simulink model "ng_pv_dynamic_dbus_p_1_sm_ng"  (Simulink 8.8)
settings: Solver=ode4  StartTime=0.0  StopTime=inf  FixedStep=0.000125  RelTol=1e-3  EnableMultiTasking=on
PreLoadFcn:
  | Ts=125e-6;Core_Num = 0; np=1; nq=1; Vmin=.9;
PostLoadFcn:
  | Ts=125e-6;Core_Num = 0; np=1; nq=1; Vmin=.9;
InitFcn:
  | Ts=125e-6;Core_Num = 0; np=1; nq=1; Vmin=.9;
undefined symbols (not defined in the file or in its folder): another_event_name, DiscIntNeverNeededParam, I, j, Left, my_event_name, Right, type, V, X
libraries: powerlib x316, simulink_extras x78, powerlib_meascontrol x47, ssn_lib x9, opal_lib x5, powerlib_extras x3, simulink x3, artemis x1, rtio_opalrt_ml605ex1 x1, rtlab x1, rtio_spectracom x1
(part 6 of 11)

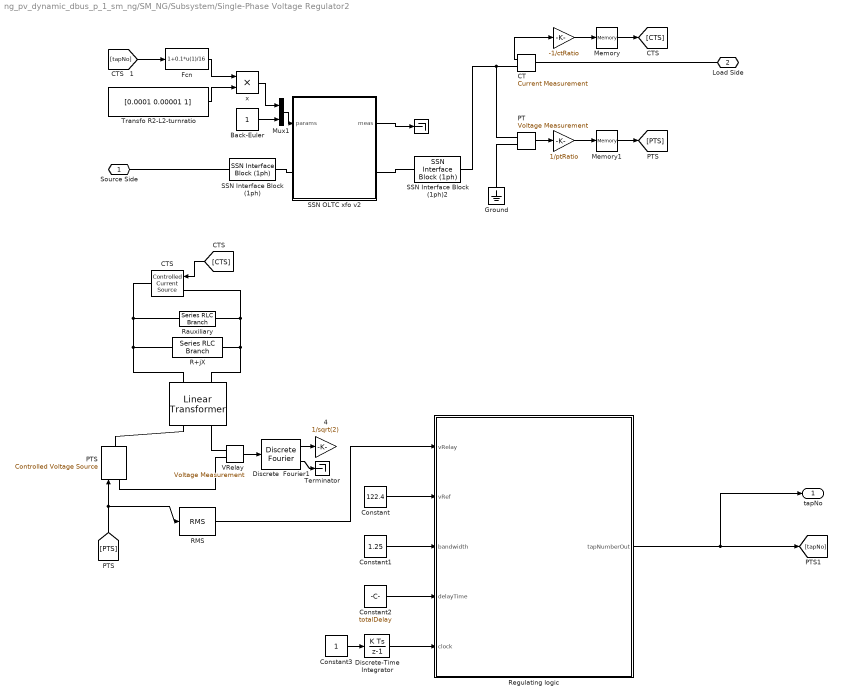
== system ng_pv_dynamic_dbus_p_1_sm_ng/SM_NG/Subsystem/Single-Phase Voltage Regulator2 ==
  " " : Gain  Gain=-1/ctRatio
  "   " : Terminator
  "    " : Gain  Gain=1/ptRatio
  "        " : powerlib/Elements/Linear Transformer  UNITS=SI  NominalPower=[pNom fNom]  winding1=[vNom/ptRatio 1.152e-007 1.2223e-008]  winding2=[vNom/ptRatio 1.152e-007 1.2223e-008]  ThreeWindings=off  winding3=[3.15e+005 0.7938 0.084225]  RmLm=[1.3824e+005 366.69]  Measurements=None  DataType=on
  "    4" : Gain  Gain=1/sqrt(2)
  Back-Euler : Constant
  CT : powerlib/Measurements/Current Measurement  PhasorSimulation=off  OutputType=Complex  PSBequivalent=0
  "CTS  " : powerlib/Electrical Sources/Controlled Current Source  Initialize=on  Source_Type=AC  Amplitude=0  Phase=0  Frequency=0  Measurements=None
  Constant : Constant  Value=122.4
  Constant1 : Constant  Value=1.25
  Constant2 : Constant  Value=totalDelay
  Constant3 : Constant
  Discrete  Fourier1 : powerlib_extras/Discrete Measurements/Discrete  Fourier  Freq=fNom  n=1  Par_Init=[0 0]  Ts=Ts
  Discrete-Time Integrator : DiscreteIntegrator  SampleTime=-1  ICPrevOutput=DiscIntNeverNeededParam  ICPrevScaledInput=DiscIntNeverNeededParam
  Fcn : Fcn  Expr=1+0.1*u(1)/16
  Ground : powerlib/Elements/Ground  LConnTagsString=a
  Memory : Memory
  Memory1 : Memory
  Mux1 : Mux  Inputs=2
  PT : powerlib/Measurements/Voltage Measurement  PhasorSimulation=off  OutputType=Complex  PSBequivalent=0
  "PTS  " : powerlib/Electrical Sources/Controlled Voltage Source  Initialize=on  Source_Type=AC  Amplitude=0  Phase=0  Frequency=0  Measurements=None
  R+jX : powerlib/Elements/Series RLC Branch  LConnTagsString=__new0  RConnTagsString=__new0  BranchType=RL  Resistance=r  Inductance=x / (2*pi*fNom)  SetiL0=off  InitialCurrent=0  Capacitance=1e-6  Setx0=off  InitialVoltage=0  Measurements=None
  RMS : powerlib_meascontrol/Measurements/RMS  TrueRMS=on  Freq=60  RMSInit=120  Ts=Ts
  Rauxiliary : powerlib/Elements/Series RLC Branch  LConnTagsString=__new0  RConnTagsString=__new0  BranchType=R  Resistance=1e3  Inductance=1.6 / (120*pi)  SetiL0=off  InitialCurrent=0  Capacitance=1e-6  Setx0=off  InitialVoltage=0  Measurements=None
  Regulating logic : MATLAB Function  TreatAsAtomicUnit=on
  SSN Interface Block (1ph) : ssn_lib/SSN Interface Block (1ph)  nb_phase=1  nb_port=2  p1_type=V-type(Left)  p2_type=X-type(Right)  p3_type=V-type(Left)  p4_type=V-type(Left)  p5_type=V-type(Left)  p6_type=V-type(Left)  p7_type=V-type(Left)  p8_type=V-type(Left)  p9_type=V-type(Left)  p10_type=V-type(Left)  p11_type=V-type(Left)  p12_type=V-type(Left)  p13_type=V-type(Left)  p14_type=V-type(Left)  p15_type=V-type(Left)  p16_type=V-type(Left)  I_port_shunt_resistance=1e9
  SSN Interface Block (1ph)2 : ssn_lib/SSN Interface Block (1ph)  nb_phase=1  nb_port=2  p1_type=X-type(Left)  p2_type=I-type(Right)  p3_type=X-type(Left)  p4_type=V-type (Right)  p5_type=V-type(Left)  p6_type=V-type(Left)  p7_type=V-type(Left)  p8_type=V-type(Left)  p9_type=V-type(Left)  p10_type=V-type(Left)  p11_type=V-type(Left)  p12_type=V-type(Left)  p13_type=V-type(Left)  p14_type=V-type(Left)  p15_type=V-type(Left)  p16_type=V-type(Left)  I_port_shunt_resistance=1e9
  SSN OLTC xfo v2 : Subsystem  AncestorBlock=artemis/SSN/SSN OLTC/SSN OLTC xfo v2  mask(Norton-Type External Nodal Subsystem){nnode=2, taggg=081xa09bxd1beaba51875, conntype=2 ports, RLpri=[1e-4 1e-5], Rcore=10000, ensat=on, Lcore=1000, Lsat=1000, phisat=1e8, Ts=Ts}
      mask prompts: nnode "Number of Electric nodes"; taggg "Unique Tag Identifier (automatic)"; conntype "Connection type"; RLpri "Primary winding resistance and inductance ([Ohms H])"; Rcore "Core Resistance (Ohms)"; ensat "Enable Saturation"; Lcore "Unsaturated magnetisation inductance (H)"; Lsat "Saturated magnetisation inductance (H)"; phisat "Flux saturation threshold (Weber)"; Ts "Sample Time (s)"
      mask help:
      | Continuously-variable On-Load Tapped Transformer (OLTC) (SSN Custom model)
      |
      | This block implements a 2 winding OLTC saturable transformer in SSN.
      | The model has a variable secondary inductance and resistance as well as turn-ratio.
      | The secondary winding is on the side marked with 'TAP'
      |
      | Mask parameters:
      |    Unique Tag Identifier: unique tag required by SSN to recknonize SSN external models
      |    Primary winding resistance and inductance ([Ohms H])
      |    Core Resistance (Ohms)
      |    Unsaturated magnetisation inductance (H): unsaturated core magnetization inductance
      |    Saturated magnetisation inductance (H): local inductance of the core in the saturated region
      |    Flux saturation threshold (Weber): flux saturation point
      |
      | Signal parameters:
      |
      | Signal inputs:
      |    1st sig: secondary winding resistance (Ohms)
      |    2nd sig: secondary winding inductance (H)
      |    3rd sig: transformer turn ratio k (V_secondary_tapped=k*V_primary)
      |    4th sig:  when set to 1, uses the Backward Euler method for solver. This can be used dynamically during simulation for example to damp numerical oscillations after switching events or after tap changes.
      |
      | Signals ouputs:
      |    1st signal: primary input current (A)
      |    2nd signal: secondary winding current (A)
      |    3rd signal: transformer flux (Wb)
      |
      | Saturation characteristic:
      |          flux
      |             ^              2
      |             |      1       *   <--- slope between point1 and point2 is Lsaturated
      |  phisat  |-----*  <---  this is the knee of flux=f(imag)
      |             |
      |             |
      |             |  <-----slope between origin and point1 is Lunsaturated
      |             *-------------------> imag
      mask init: same as ng_pv_dynamic_dbus_p_1_sm_ng/SM_NG/Subsystem/Single-Phase Voltage Regulator1/SSN OLTC xfo v2
      settings: CopyFcn=|
      | str=tempname;
      | str=strrep(str(end-20:end),'_','x');
      | set_param(gcb,'taggg',str);
      | set_param(gcb,'LinkStatus','inactive');
      mask Help: eval('open SSN_OLTC.pdf;');
      mask TypeOptions conntype: 4 ports | 3 ports (primary grounded) | 3 ports (tapped secondary grounded) | 2 ports
      mask Callback conntype:
      | bloc=gcb;
      | conntyp=get_param(bloc,'conntype');
      | nn=fts6_xfo_port_cb(bloc,conntyp);
      | set_param(bloc,'nnode',nn);
      mask Display:
      | plot(a1,a2,a3,a4,b1,b2,b3,b4,c1,c2,c3,c4,c5,c6,c7,c8,c9,c10,c11,c12,c13,c14,c15,c16);
      | color('blue');
      | plot(d1,d2,d3,d4,d5,d6,d7,d8,d9,d10);
  Terminator : Terminator
  Transfo R2-L2-turnratio : Constant  Value=[0.0001 0.00001 1]
  VRelay : powerlib/Measurements/Voltage Measurement  PhasorSimulation=off  OutputType=Complex  PSBequivalent=0
  x : Product  RndMeth=Zero
  Source Side : PMIOPort  Port=1  Side=Left
  Load Side : PMIOPort  Port=2  Side=Right
  tapNo : Outport
  wires:
  CT/1 -> " "/1
  " "/1 -> Memory/1
  PT/1 -> "    "/1
  "    "/1 -> Memory1/1
  [CTS] -> "CTS  "/1
  [PTS] -> RMS/1, "PTS  "/1
  VRelay/1 -> Discrete  Fourier1/1
  Discrete  Fourier1/1 -> "    4"/1
  Discrete-Time Integrator/1 -> Regulating logic/5(clock)
  Regulating logic/1(tapNumberOut) -> [tapNo], tapNo/1
  Constant/1 -> Regulating logic/2(vRef)
  Constant1/1 -> Regulating logic/3(bandwidth)
  Constant2/1 -> Regulating logic/4(delayTime)
  Memory/1 -> [CTS]
  Memory1/1 -> [PTS]
  Discrete  Fourier1/2 -> Terminator/1
  Back-Euler/1 -> Mux1/2
  Transfo R2-L2-turnratio/1 -> x/2
  x/1 -> Mux1/1
  Fcn/1 -> x/1
  [tapNo] -> Fcn/1
  Constant3/1 -> Discrete-Time Integrator/1
  RMS/1 -> Regulating logic/1(vRelay)
  Mux1/1 -> SSN OLTC xfo v2/1(params)
  SSN OLTC xfo v2/1(meas) -> "   "/1
  connections:
  R+jX/LConn1 -- "        "/LConn1 -- "CTS  "/RConn1 -- Rauxiliary/LConn1
  R+jX/RConn1 -- "        "/LConn2 -- "CTS  "/LConn1 -- Rauxiliary/RConn1
  "PTS  "/RConn1 -- "        "/RConn1
  "        "/RConn2 -- VRelay/LConn1
  PT/LConn1 -- CT/RConn1 -- SSN Interface Block (1ph)2/RConn1
  PT/LConn2 -- Ground/LConn1
  VRelay/LConn2 -- "PTS  "/LConn1
  Load Side/RConn1 -- CT/LConn1
  SSN Interface Block (1ph)/RConn1 -- SSN OLTC xfo v2/LConn1
  SSN Interface Block (1ph)2/LConn1 -- SSN OLTC xfo v2/RConn1
  SSN Interface Block (1ph)/LConn1 -- Source Side/RConn1

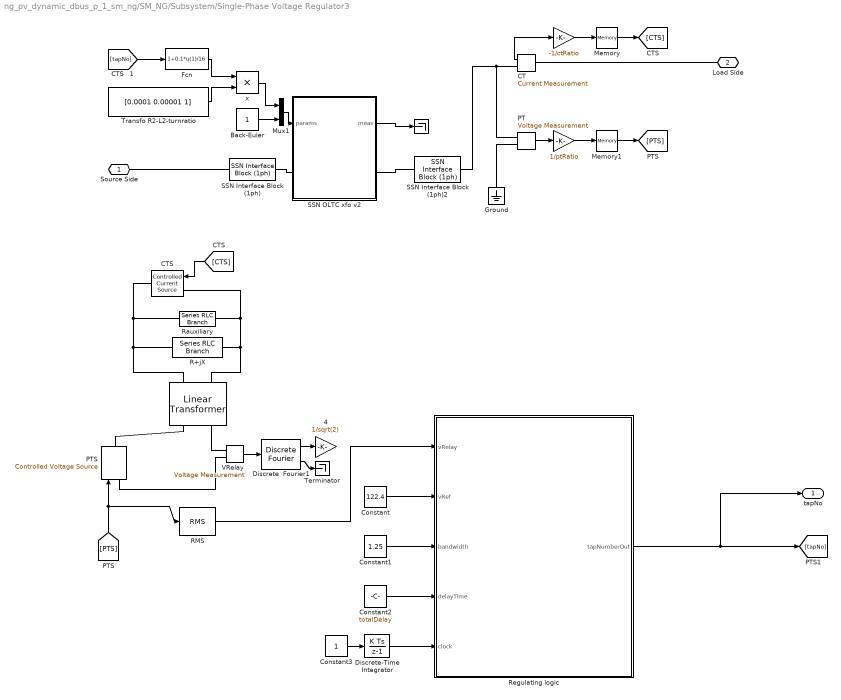
== system ng_pv_dynamic_dbus_p_1_sm_ng/SM_NG/Subsystem/Single-Phase Voltage Regulator3 ==
  " " : Gain  Gain=-1/ctRatio
  "   " : Terminator
  "    " : Gain  Gain=1/ptRatio
  "        " : powerlib/Elements/Linear Transformer  UNITS=SI  NominalPower=[pNom fNom]  winding1=[vNom/ptRatio 1.152e-007 1.2223e-008]  winding2=[vNom/ptRatio 1.152e-007 1.2223e-008]  ThreeWindings=off  winding3=[3.15e+005 0.7938 0.084225]  RmLm=[1.3824e+005 366.69]  Measurements=None  DataType=on
  "    4" : Gain  Gain=1/sqrt(2)
  Back-Euler : Constant
  CT : powerlib/Measurements/Current Measurement  PhasorSimulation=off  OutputType=Complex  PSBequivalent=0
  "CTS  " : powerlib/Electrical Sources/Controlled Current Source  Initialize=on  Source_Type=AC  Amplitude=0  Phase=0  Frequency=0  Measurements=None
  Constant : Constant  Value=122.4
  Constant1 : Constant  Value=1.25
  Constant2 : Constant  Value=totalDelay
  Constant3 : Constant
  Discrete  Fourier1 : powerlib_extras/Discrete Measurements/Discrete  Fourier  Freq=fNom  n=1  Par_Init=[0 0]  Ts=Ts
  Discrete-Time Integrator : DiscreteIntegrator  SampleTime=-1  ICPrevOutput=DiscIntNeverNeededParam  ICPrevScaledInput=DiscIntNeverNeededParam
  Fcn : Fcn  Expr=1+0.1*u(1)/16
  Ground : powerlib/Elements/Ground  LConnTagsString=a
  Memory : Memory
  Memory1 : Memory
  Mux1 : Mux  Inputs=2
  PT : powerlib/Measurements/Voltage Measurement  PhasorSimulation=off  OutputType=Complex  PSBequivalent=0
  "PTS  " : powerlib/Electrical Sources/Controlled Voltage Source  Initialize=on  Source_Type=AC  Amplitude=0  Phase=0  Frequency=0  Measurements=None
  R+jX : powerlib/Elements/Series RLC Branch  LConnTagsString=__new0  RConnTagsString=__new0  BranchType=RL  Resistance=r  Inductance=x / (2*pi*fNom)  SetiL0=off  InitialCurrent=0  Capacitance=1e-6  Setx0=off  InitialVoltage=0  Measurements=None
  RMS : powerlib_meascontrol/Measurements/RMS  TrueRMS=on  Freq=60  RMSInit=120  Ts=Ts
  Rauxiliary : powerlib/Elements/Series RLC Branch  LConnTagsString=__new0  RConnTagsString=__new0  BranchType=R  Resistance=1e3  Inductance=1.6 / (120*pi)  SetiL0=off  InitialCurrent=0  Capacitance=1e-6  Setx0=off  InitialVoltage=0  Measurements=None
  Regulating logic : MATLAB Function  TreatAsAtomicUnit=on
  SSN Interface Block (1ph) : ssn_lib/SSN Interface Block (1ph)  nb_phase=1  nb_port=2  p1_type=V-type(Left)  p2_type=X-type(Right)  p3_type=V-type(Left)  p4_type=V-type(Left)  p5_type=V-type(Left)  p6_type=V-type(Left)  p7_type=V-type(Left)  p8_type=V-type(Left)  p9_type=V-type(Left)  p10_type=V-type(Left)  p11_type=V-type(Left)  p12_type=V-type(Left)  p13_type=V-type(Left)  p14_type=V-type(Left)  p15_type=V-type(Left)  p16_type=V-type(Left)  I_port_shunt_resistance=1e9
  SSN Interface Block (1ph)2 : ssn_lib/SSN Interface Block (1ph)  nb_phase=1  nb_port=2  p1_type=X-type(Left)  p2_type=I-type(Right)  p3_type=X-type(Left)  p4_type=V-type (Right)  p5_type=V-type(Left)  p6_type=V-type(Left)  p7_type=V-type(Left)  p8_type=V-type(Left)  p9_type=V-type(Left)  p10_type=V-type(Left)  p11_type=V-type(Left)  p12_type=V-type(Left)  p13_type=V-type(Left)  p14_type=V-type(Left)  p15_type=V-type(Left)  p16_type=V-type(Left)  I_port_shunt_resistance=1e9
  SSN OLTC xfo v2 : Subsystem  AncestorBlock=artemis/SSN/SSN OLTC/SSN OLTC xfo v2  mask(Norton-Type External Nodal Subsystem){nnode=2, taggg=e32xb02fxc50b2a824a30, conntype=2 ports, RLpri=[1e-4 1e-5], Rcore=10000, ensat=on, Lcore=1000, Lsat=1000, phisat=1e8, Ts=Ts}
      mask prompts: nnode "Number of Electric nodes"; taggg "Unique Tag Identifier (automatic)"; conntype "Connection type"; RLpri "Primary winding resistance and inductance ([Ohms H])"; Rcore "Core Resistance (Ohms)"; ensat "Enable Saturation"; Lcore "Unsaturated magnetisation inductance (H)"; Lsat "Saturated magnetisation inductance (H)"; phisat "Flux saturation threshold (Weber)"; Ts "Sample Time (s)"
      mask help:
      | Continuously-variable On-Load Tapped Transformer (OLTC) (SSN Custom model)
      |
      | This block implements a 2 winding OLTC saturable transformer in SSN.
      | The model has a variable secondary inductance and resistance as well as turn-ratio.
      | The secondary winding is on the side marked with 'TAP'
      |
      | Mask parameters:
      |    Unique Tag Identifier: unique tag required by SSN to recknonize SSN external models
      |    Primary winding resistance and inductance ([Ohms H])
      |    Core Resistance (Ohms)
      |    Unsaturated magnetisation inductance (H): unsaturated core magnetization inductance
      |    Saturated magnetisation inductance (H): local inductance of the core in the saturated region
      |    Flux saturation threshold (Weber): flux saturation point
      |
      | Signal parameters:
      |
      | Signal inputs:
      |    1st sig: secondary winding resistance (Ohms)
      |    2nd sig: secondary winding inductance (H)
      |    3rd sig: transformer turn ratio k (V_secondary_tapped=k*V_primary)
      |    4th sig:  when set to 1, uses the Backward Euler method for solver. This can be used dynamically during simulation for example to damp numerical oscillations after switching events or after tap changes.
      |
      | Signals ouputs:
      |    1st signal: primary input current (A)
      |    2nd signal: secondary winding current (A)
      |    3rd signal: transformer flux (Wb)
      |
      | Saturation characteristic:
      |          flux
      |             ^              2
      |             |      1       *   <--- slope between point1 and point2 is Lsaturated
      |  phisat  |-----*  <---  this is the knee of flux=f(imag)
      |             |
      |             |
      |             |  <-----slope between origin and point1 is Lunsaturated
      |             *-------------------> imag
      mask init: same as ng_pv_dynamic_dbus_p_1_sm_ng/SM_NG/Subsystem/Single-Phase Voltage Regulator1/SSN OLTC xfo v2
      settings: CopyFcn=|
      | str=tempname;
      | str=strrep(str(end-20:end),'_','x');
      | set_param(gcb,'taggg',str);
      | set_param(gcb,'LinkStatus','inactive');
      mask Help: eval('open SSN_OLTC.pdf;');
      mask TypeOptions conntype: 4 ports | 3 ports (primary grounded) | 3 ports (tapped secondary grounded) | 2 ports
      mask Callback conntype:
      | bloc=gcb;
      | conntyp=get_param(bloc,'conntype');
      | nn=fts6_xfo_port_cb(bloc,conntyp);
      | set_param(bloc,'nnode',nn);
      mask Display:
      | plot(a1,a2,a3,a4,b1,b2,b3,b4,c1,c2,c3,c4,c5,c6,c7,c8,c9,c10,c11,c12,c13,c14,c15,c16);
      | color('blue');
      | plot(d1,d2,d3,d4,d5,d6,d7,d8,d9,d10);
  Terminator : Terminator
  Transfo R2-L2-turnratio : Constant  Value=[0.0001 0.00001 1]
  VRelay : powerlib/Measurements/Voltage Measurement  PhasorSimulation=off  OutputType=Complex  PSBequivalent=0
  x : Product  RndMeth=Zero
  Source Side : PMIOPort  Port=1  Side=Left
  Load Side : PMIOPort  Port=2  Side=Right
  tapNo : Outport
  wires:
  CT/1 -> " "/1
  " "/1 -> Memory/1
  PT/1 -> "    "/1
  "    "/1 -> Memory1/1
  [CTS] -> "CTS  "/1
  [PTS] -> RMS/1, "PTS  "/1
  VRelay/1 -> Discrete  Fourier1/1
  Discrete  Fourier1/1 -> "    4"/1
  Discrete-Time Integrator/1 -> Regulating logic/5(clock)
  Regulating logic/1(tapNumberOut) -> [tapNo], tapNo/1
  Constant/1 -> Regulating logic/2(vRef)
  Constant1/1 -> Regulating logic/3(bandwidth)
  Constant2/1 -> Regulating logic/4(delayTime)
  Memory/1 -> [CTS]
  Memory1/1 -> [PTS]
  Discrete  Fourier1/2 -> Terminator/1
  Back-Euler/1 -> Mux1/2
  Transfo R2-L2-turnratio/1 -> x/2
  x/1 -> Mux1/1
  Fcn/1 -> x/1
  [tapNo] -> Fcn/1
  Constant3/1 -> Discrete-Time Integrator/1
  RMS/1 -> Regulating logic/1(vRelay)
  Mux1/1 -> SSN OLTC xfo v2/1(params)
  SSN OLTC xfo v2/1(meas) -> "   "/1
  connections:
  R+jX/LConn1 -- "        "/LConn1 -- "CTS  "/RConn1 -- Rauxiliary/LConn1
  R+jX/RConn1 -- "        "/LConn2 -- "CTS  "/LConn1 -- Rauxiliary/RConn1
  "PTS  "/RConn1 -- "        "/RConn1
  "        "/RConn2 -- VRelay/LConn1
  PT/LConn1 -- CT/RConn1 -- SSN Interface Block (1ph)2/RConn1
  PT/LConn2 -- Ground/LConn1
  VRelay/LConn2 -- "PTS  "/LConn1
  Load Side/RConn1 -- CT/LConn1
  SSN Interface Block (1ph)/RConn1 -- SSN OLTC xfo v2/LConn1
  SSN Interface Block (1ph)2/LConn1 -- SSN OLTC xfo v2/RConn1
  SSN Interface Block (1ph)/LConn1 -- Source Side/RConn1

== system ng_pv_dynamic_dbus_p_1_sm_ng/SM_NG/rtlab_send_subsystem/Subsystem1 ==
  In1 : Inport
  In2 : Inport  Port=2
  In3 : Inport  Port=3
  In4 : Inport  Port=4
  Mux : Mux
  Send1 : opal_lib/Communication/OpSendToNT  Acqu_group=1
  wires:
  Mux/1 -> Send1/1
  In1/1 -> Mux/1
  In2/1 -> Mux/2
  In3/1 -> Mux/3
  In4/1 -> Mux/4

== system ng_pv_dynamic_dbus_p_1_sm_ng/SM_NG/rtlab_send_subsystem/Subsystem3 ==
  In1 : Inport
  Mux : Mux  Inputs=1
  Send3 : opal_lib/Communication/OpSend_rt  dest=3  priority2=0  st=0.000125
  wires:
  Mux/1 -> Send3/1
  In1/1 -> Mux/1

== system ng_pv_dynamic_dbus_p_1_sm_ng/SM_NG/rtlab_send_subsystem/Subsystem4 ==
  In1 : Inport
  In2 : Inport  Port=2
  Mux : Mux  Inputs=2
  Send4 : opal_lib/Communication/OpSend_rt  dest=4  priority2=0  st=0.000125
  wires:
  Mux/1 -> Send4/1
  In1/1 -> Mux/1
  In2/1 -> Mux/2

== system ng_pv_dynamic_dbus_p_1_sm_ng/SM_NG/zzzOpComm/busStruct ==
  In1 : Inport
  Sub1 : Subsystem
  Out1 : Outport
  wires:
  Sub1/1(out) -> Out1/1
  In1/1 -> Sub1/1(in)

== system ng_pv_dynamic_dbus_p_1_sm_ng/SM_NG/Dynamic Load BCDC1/Single-Phase Dynamic Load1/model ==
  v : Inport
  PQ : Inport  Port=2
  Break  Alg. Loop1 : Subsystem
  Complex to Magnitude-Angle : ComplexToMagnitudeAngle
  Complex to Real-Imag1 : ComplexToRealImag
  Constant : Constant
  Demux : Demux  Outputs=2
  Divide : Product  Inputs=**
  Gain : Gain  Gain=1.0114
  IC1 : InitialCondition
  IC2 : InitialCondition
  Magnitude-Angle to Complex : MagnitudeAngleToComplex
  PLL : Subsystem  mask{freq=fnom}
      mask prompts: freq "Initial frequency (Hz)"
  Positive Sequence  current : Subsystem
  RMS1 : powerlib_meascontrol/Measurements/RMS  TrueRMS=on  Freq=fnom  RMSInit=1  Ts=0
  Real-Imag to Complex : RealImagToComplex
  Real-Imag to Complex1 : RealImagToComplex
  Sum : Sum
  Transfer Fcn1 : TransferFcn  Numerator=[1 290.1]  Denominator=[1 298.8]
  Trigonometric Function1 : Trigonometry
  V> pu : Gain  Gain=1/Vbase/sqrt(3)  SaturateOnIntegerOverflow=on  OutDataTypeStr=Inherit: Same as input  ParamDataTypeStr=Inherit: Same as input
  V> pu1 : Gain  Gain=sqrt(2)  SaturateOnIntegerOverflow=on  OutDataTypeStr=Inherit: Same as input  ParamDataTypeStr=Inherit: Same as input
  i : Outport
  wires:
  V> pu/1 -> PLL/1(v (pu)), V> pu1/1
  Real-Imag to Complex/1 -> Positive Sequence  current/1(V1(pu))
  PQ/1 -> Demux/1
  Demux/1 -> Real-Imag to Complex1/1
  Demux/2 -> Real-Imag to Complex1/2
  Real-Imag to Complex1/1 -> Positive Sequence  current/2(S_ext)
  Complex to Real-Imag1/1 -> Real-Imag to Complex/1
  Complex to Real-Imag1/2 -> Real-Imag to Complex/2
  Magnitude-Angle to Complex/1 -> Complex to Real-Imag1/1
  Constant/1 -> PLL/2(freq (pu))
  PLL/1(alpha (rad)) -> Magnitude-Angle to Complex/2
  Complex to Magnitude-Angle/2 -> Sum/2
  PLL/2(wt) -> Sum/1
  Sum/1 -> Trigonometric Function1/1
  Trigonometric Function1/1 -> Divide/2
  Complex to Magnitude-Angle/1 -> Divide/1
  RMS1/1 -> IC1/1
  V> pu1/1 -> RMS1/1
  v/1 -> IC2/1
  Positive Sequence  current/1(I1(A)) -> Break  Alg. Loop1/1(In)
  Break  Alg. Loop1/1(Out) -> Complex to Magnitude-Angle/1
  IC1/1 -> Magnitude-Angle to Complex/1
  IC2/1 -> V> pu/1
  Transfer Fcn1/1 -> Gain/1
  Gain/1 -> i/1
  Divide/1 -> Transfer Fcn1/1

== system ng_pv_dynamic_dbus_p_1_sm_ng/SM_NG/Dynamic Load BCDC1/Single-Phase Dynamic Load2/model ==
  v : Inport
  PQ : Inport  Port=2
  Break  Alg. Loop1 : Subsystem
  Complex to Magnitude-Angle : ComplexToMagnitudeAngle
  Complex to Real-Imag1 : ComplexToRealImag
  Constant : Constant
  Demux : Demux  Outputs=2
  Divide : Product  Inputs=**
  Gain : Gain  Gain=1.0114
  IC1 : InitialCondition
  IC2 : InitialCondition
  Magnitude-Angle to Complex : MagnitudeAngleToComplex
  PLL : Subsystem  mask{freq=fnom}
      mask prompts: freq "Initial frequency (Hz)"
  Positive Sequence  current : Subsystem
  RMS1 : powerlib_meascontrol/Measurements/RMS  TrueRMS=on  Freq=fnom  RMSInit=1  Ts=0
  Real-Imag to Complex : RealImagToComplex
  Real-Imag to Complex1 : RealImagToComplex
  Sum : Sum
  Transfer Fcn1 : TransferFcn  Numerator=[1 290.1]  Denominator=[1 298.8]
  Trigonometric Function1 : Trigonometry
  V> pu : Gain  Gain=1/Vbase/sqrt(3)  SaturateOnIntegerOverflow=on  OutDataTypeStr=Inherit: Same as input  ParamDataTypeStr=Inherit: Same as input
  V> pu1 : Gain  Gain=sqrt(2)  SaturateOnIntegerOverflow=on  OutDataTypeStr=Inherit: Same as input  ParamDataTypeStr=Inherit: Same as input
  i : Outport
  wires:
  V> pu/1 -> PLL/1(v (pu)), V> pu1/1
  Real-Imag to Complex/1 -> Positive Sequence  current/1(V1(pu))
  PQ/1 -> Demux/1
  Demux/1 -> Real-Imag to Complex1/1
  Demux/2 -> Real-Imag to Complex1/2
  Real-Imag to Complex1/1 -> Positive Sequence  current/2(S_ext)
  Complex to Real-Imag1/1 -> Real-Imag to Complex/1
  Complex to Real-Imag1/2 -> Real-Imag to Complex/2
  Magnitude-Angle to Complex/1 -> Complex to Real-Imag1/1
  Constant/1 -> PLL/2(freq (pu))
  PLL/1(alpha (rad)) -> Magnitude-Angle to Complex/2
  Complex to Magnitude-Angle/2 -> Sum/2
  PLL/2(wt) -> Sum/1
  Sum/1 -> Trigonometric Function1/1
  Trigonometric Function1/1 -> Divide/2
  Complex to Magnitude-Angle/1 -> Divide/1
  RMS1/1 -> IC1/1
  V> pu1/1 -> RMS1/1
  v/1 -> IC2/1
  Positive Sequence  current/1(I1(A)) -> Break  Alg. Loop1/1(In)
  Break  Alg. Loop1/1(Out) -> Complex to Magnitude-Angle/1
  IC1/1 -> Magnitude-Angle to Complex/1
  IC2/1 -> V> pu/1
  Transfer Fcn1/1 -> Gain/1
  Gain/1 -> i/1
  Divide/1 -> Transfer Fcn1/1

== system ng_pv_dynamic_dbus_p_1_sm_ng/SM_NG/Dynamic Load BCDC1/Single-Phase Dynamic Load9/model ==
  v : Inport
  PQ : Inport  Port=2
  Break  Alg. Loop1 : Subsystem
  Complex to Magnitude-Angle : ComplexToMagnitudeAngle
  Complex to Real-Imag1 : ComplexToRealImag
  Constant : Constant
  Demux : Demux  Outputs=2
  Divide : Product  Inputs=**
  Gain : Gain  Gain=1.0114
  IC1 : InitialCondition
  IC2 : InitialCondition
  Magnitude-Angle to Complex : MagnitudeAngleToComplex
  PLL : Subsystem  mask{freq=fnom}
      mask prompts: freq "Initial frequency (Hz)"
  Positive Sequence  current : Subsystem
  RMS1 : powerlib_meascontrol/Measurements/RMS  TrueRMS=on  Freq=fnom  RMSInit=1  Ts=0
  Real-Imag to Complex : RealImagToComplex
  Real-Imag to Complex1 : RealImagToComplex
  Sum : Sum
  Transfer Fcn1 : TransferFcn  Numerator=[1 290.1]  Denominator=[1 298.8]
  Trigonometric Function1 : Trigonometry
  V> pu : Gain  Gain=1/Vbase/sqrt(3)  SaturateOnIntegerOverflow=on  OutDataTypeStr=Inherit: Same as input  ParamDataTypeStr=Inherit: Same as input
  V> pu1 : Gain  Gain=sqrt(2)  SaturateOnIntegerOverflow=on  OutDataTypeStr=Inherit: Same as input  ParamDataTypeStr=Inherit: Same as input
  i : Outport
  wires:
  V> pu/1 -> PLL/1(v (pu)), V> pu1/1
  Real-Imag to Complex/1 -> Positive Sequence  current/1(V1(pu))
  PQ/1 -> Demux/1
  Demux/1 -> Real-Imag to Complex1/1
  Demux/2 -> Real-Imag to Complex1/2
  Real-Imag to Complex1/1 -> Positive Sequence  current/2(S_ext)
  Complex to Real-Imag1/1 -> Real-Imag to Complex/1
  Complex to Real-Imag1/2 -> Real-Imag to Complex/2
  Magnitude-Angle to Complex/1 -> Complex to Real-Imag1/1
  Constant/1 -> PLL/2(freq (pu))
  PLL/1(alpha (rad)) -> Magnitude-Angle to Complex/2
  Complex to Magnitude-Angle/2 -> Sum/2
  PLL/2(wt) -> Sum/1
  Sum/1 -> Trigonometric Function1/1
  Trigonometric Function1/1 -> Divide/2
  Complex to Magnitude-Angle/1 -> Divide/1
  RMS1/1 -> IC1/1
  V> pu1/1 -> RMS1/1
  v/1 -> IC2/1
  Positive Sequence  current/1(I1(A)) -> Break  Alg. Loop1/1(In)
  Break  Alg. Loop1/1(Out) -> Complex to Magnitude-Angle/1
  IC1/1 -> Magnitude-Angle to Complex/1
  IC2/1 -> V> pu/1
  Transfer Fcn1/1 -> Gain/1
  Gain/1 -> i/1
  Divide/1 -> Transfer Fcn1/1

== system ng_pv_dynamic_dbus_p_1_sm_ng/SM_NG/Dynamic Load BCDC2/Single-Phase Dynamic Load1/model ==
  v : Inport
  PQ : Inport  Port=2
  Break  Alg. Loop1 : Subsystem
  Complex to Magnitude-Angle : ComplexToMagnitudeAngle
  Complex to Real-Imag1 : ComplexToRealImag
  Constant : Constant
  Demux : Demux  Outputs=2
  Divide : Product  Inputs=**
  Gain : Gain  Gain=1.0114
  IC1 : InitialCondition
  IC2 : InitialCondition
  Magnitude-Angle to Complex : MagnitudeAngleToComplex
  PLL : Subsystem  mask{freq=fnom}
      mask prompts: freq "Initial frequency (Hz)"
  Positive Sequence  current : Subsystem
  RMS1 : powerlib_meascontrol/Measurements/RMS  TrueRMS=on  Freq=fnom  RMSInit=1  Ts=0
  Real-Imag to Complex : RealImagToComplex
  Real-Imag to Complex1 : RealImagToComplex
  Sum : Sum
  Transfer Fcn1 : TransferFcn  Numerator=[1 290.1]  Denominator=[1 298.8]
  Trigonometric Function1 : Trigonometry
  V> pu : Gain  Gain=1/Vbase/sqrt(3)  SaturateOnIntegerOverflow=on  OutDataTypeStr=Inherit: Same as input  ParamDataTypeStr=Inherit: Same as input
  V> pu1 : Gain  Gain=sqrt(2)  SaturateOnIntegerOverflow=on  OutDataTypeStr=Inherit: Same as input  ParamDataTypeStr=Inherit: Same as input
  i : Outport
  wires:
  V> pu/1 -> PLL/1(v (pu)), V> pu1/1
  Real-Imag to Complex/1 -> Positive Sequence  current/1(V1(pu))
  PQ/1 -> Demux/1
  Demux/1 -> Real-Imag to Complex1/1
  Demux/2 -> Real-Imag to Complex1/2
  Real-Imag to Complex1/1 -> Positive Sequence  current/2(S_ext)
  Complex to Real-Imag1/1 -> Real-Imag to Complex/1
  Complex to Real-Imag1/2 -> Real-Imag to Complex/2
  Magnitude-Angle to Complex/1 -> Complex to Real-Imag1/1
  Constant/1 -> PLL/2(freq (pu))
  PLL/1(alpha (rad)) -> Magnitude-Angle to Complex/2
  Complex to Magnitude-Angle/2 -> Sum/2
  PLL/2(wt) -> Sum/1
  Sum/1 -> Trigonometric Function1/1
  Trigonometric Function1/1 -> Divide/2
  Complex to Magnitude-Angle/1 -> Divide/1
  RMS1/1 -> IC1/1
  V> pu1/1 -> RMS1/1
  v/1 -> IC2/1
  Positive Sequence  current/1(I1(A)) -> Break  Alg. Loop1/1(In)
  Break  Alg. Loop1/1(Out) -> Complex to Magnitude-Angle/1
  IC1/1 -> Magnitude-Angle to Complex/1
  IC2/1 -> V> pu/1
  Transfer Fcn1/1 -> Gain/1
  Gain/1 -> i/1
  Divide/1 -> Transfer Fcn1/1

== system ng_pv_dynamic_dbus_p_1_sm_ng/SM_NG/Dynamic Load BCDC2/Single-Phase Dynamic Load2/model ==
  v : Inport
  PQ : Inport  Port=2
  Break  Alg. Loop1 : Subsystem
  Complex to Magnitude-Angle : ComplexToMagnitudeAngle
  Complex to Real-Imag1 : ComplexToRealImag
  Constant : Constant
  Demux : Demux  Outputs=2
  Divide : Product  Inputs=**
  Gain : Gain  Gain=1.0114
  IC1 : InitialCondition
  IC2 : InitialCondition
  Magnitude-Angle to Complex : MagnitudeAngleToComplex
  PLL : Subsystem  mask{freq=fnom}
      mask prompts: freq "Initial frequency (Hz)"
  Positive Sequence  current : Subsystem
  RMS1 : powerlib_meascontrol/Measurements/RMS  TrueRMS=on  Freq=fnom  RMSInit=1  Ts=0
  Real-Imag to Complex : RealImagToComplex
  Real-Imag to Complex1 : RealImagToComplex
  Sum : Sum
  Transfer Fcn1 : TransferFcn  Numerator=[1 290.1]  Denominator=[1 298.8]
  Trigonometric Function1 : Trigonometry
  V> pu : Gain  Gain=1/Vbase/sqrt(3)  SaturateOnIntegerOverflow=on  OutDataTypeStr=Inherit: Same as input  ParamDataTypeStr=Inherit: Same as input
  V> pu1 : Gain  Gain=sqrt(2)  SaturateOnIntegerOverflow=on  OutDataTypeStr=Inherit: Same as input  ParamDataTypeStr=Inherit: Same as input
  i : Outport
  wires:
  V> pu/1 -> PLL/1(v (pu)), V> pu1/1
  Real-Imag to Complex/1 -> Positive Sequence  current/1(V1(pu))
  PQ/1 -> Demux/1
  Demux/1 -> Real-Imag to Complex1/1
  Demux/2 -> Real-Imag to Complex1/2
  Real-Imag to Complex1/1 -> Positive Sequence  current/2(S_ext)
  Complex to Real-Imag1/1 -> Real-Imag to Complex/1
  Complex to Real-Imag1/2 -> Real-Imag to Complex/2
  Magnitude-Angle to Complex/1 -> Complex to Real-Imag1/1
  Constant/1 -> PLL/2(freq (pu))
  PLL/1(alpha (rad)) -> Magnitude-Angle to Complex/2
  Complex to Magnitude-Angle/2 -> Sum/2
  PLL/2(wt) -> Sum/1
  Sum/1 -> Trigonometric Function1/1
  Trigonometric Function1/1 -> Divide/2
  Complex to Magnitude-Angle/1 -> Divide/1
  RMS1/1 -> IC1/1
  V> pu1/1 -> RMS1/1
  v/1 -> IC2/1
  Positive Sequence  current/1(I1(A)) -> Break  Alg. Loop1/1(In)
  Break  Alg. Loop1/1(Out) -> Complex to Magnitude-Angle/1
  IC1/1 -> Magnitude-Angle to Complex/1
  IC2/1 -> V> pu/1
  Transfer Fcn1/1 -> Gain/1
  Gain/1 -> i/1
  Divide/1 -> Transfer Fcn1/1

== system ng_pv_dynamic_dbus_p_1_sm_ng/SM_NG/Dynamic Load BCDC2/Single-Phase Dynamic Load9/model ==
  v : Inport
  PQ : Inport  Port=2
  Break  Alg. Loop1 : Subsystem
  Complex to Magnitude-Angle : ComplexToMagnitudeAngle
  Complex to Real-Imag1 : ComplexToRealImag
  Constant : Constant
  Demux : Demux  Outputs=2
  Divide : Product  Inputs=**
  Gain : Gain  Gain=1.0114
  IC1 : InitialCondition
  IC2 : InitialCondition
  Magnitude-Angle to Complex : MagnitudeAngleToComplex
  PLL : Subsystem  mask{freq=fnom}
      mask prompts: freq "Initial frequency (Hz)"
  Positive Sequence  current : Subsystem
  RMS1 : powerlib_meascontrol/Measurements/RMS  TrueRMS=on  Freq=fnom  RMSInit=1  Ts=0
  Real-Imag to Complex : RealImagToComplex
  Real-Imag to Complex1 : RealImagToComplex
  Sum : Sum
  Transfer Fcn1 : TransferFcn  Numerator=[1 290.1]  Denominator=[1 298.8]
  Trigonometric Function1 : Trigonometry
  V> pu : Gain  Gain=1/Vbase/sqrt(3)  SaturateOnIntegerOverflow=on  OutDataTypeStr=Inherit: Same as input  ParamDataTypeStr=Inherit: Same as input
  V> pu1 : Gain  Gain=sqrt(2)  SaturateOnIntegerOverflow=on  OutDataTypeStr=Inherit: Same as input  ParamDataTypeStr=Inherit: Same as input
  i : Outport
  wires:
  V> pu/1 -> PLL/1(v (pu)), V> pu1/1
  Real-Imag to Complex/1 -> Positive Sequence  current/1(V1(pu))
  PQ/1 -> Demux/1
  Demux/1 -> Real-Imag to Complex1/1
  Demux/2 -> Real-Imag to Complex1/2
  Real-Imag to Complex1/1 -> Positive Sequence  current/2(S_ext)
  Complex to Real-Imag1/1 -> Real-Imag to Complex/1
  Complex to Real-Imag1/2 -> Real-Imag to Complex/2
  Magnitude-Angle to Complex/1 -> Complex to Real-Imag1/1
  Constant/1 -> PLL/2(freq (pu))
  PLL/1(alpha (rad)) -> Magnitude-Angle to Complex/2
  Complex to Magnitude-Angle/2 -> Sum/2
  PLL/2(wt) -> Sum/1
  Sum/1 -> Trigonometric Function1/1
  Trigonometric Function1/1 -> Divide/2
  Complex to Magnitude-Angle/1 -> Divide/1
  RMS1/1 -> IC1/1
  V> pu1/1 -> RMS1/1
  v/1 -> IC2/1
  Positive Sequence  current/1(I1(A)) -> Break  Alg. Loop1/1(In)
  Break  Alg. Loop1/1(Out) -> Complex to Magnitude-Angle/1
  IC1/1 -> Magnitude-Angle to Complex/1
  IC2/1 -> V> pu/1
  Transfer Fcn1/1 -> Gain/1
  Gain/1 -> i/1
  Divide/1 -> Transfer Fcn1/1

== system ng_pv_dynamic_dbus_p_1_sm_ng/SM_NG/Dynamic Load BCDC3/Single-Phase Dynamic Load1/model ==
  v : Inport
  PQ : Inport  Port=2
  Break  Alg. Loop1 : Subsystem
  Complex to Magnitude-Angle : ComplexToMagnitudeAngle
  Complex to Real-Imag1 : ComplexToRealImag
  Constant : Constant
  Demux : Demux  Outputs=2
  Divide : Product  Inputs=**
  Gain : Gain  Gain=1.0114
  IC1 : InitialCondition
  IC2 : InitialCondition
  Magnitude-Angle to Complex : MagnitudeAngleToComplex
  PLL : Subsystem  mask{freq=fnom}
      mask prompts: freq "Initial frequency (Hz)"
  Positive Sequence  current : Subsystem
  RMS1 : powerlib_meascontrol/Measurements/RMS  TrueRMS=on  Freq=fnom  RMSInit=1  Ts=0
  Real-Imag to Complex : RealImagToComplex
  Real-Imag to Complex1 : RealImagToComplex
  Sum : Sum
  Transfer Fcn1 : TransferFcn  Numerator=[1 290.1]  Denominator=[1 298.8]
  Trigonometric Function1 : Trigonometry
  V> pu : Gain  Gain=1/Vbase/sqrt(3)  SaturateOnIntegerOverflow=on  OutDataTypeStr=Inherit: Same as input  ParamDataTypeStr=Inherit: Same as input
  V> pu1 : Gain  Gain=sqrt(2)  SaturateOnIntegerOverflow=on  OutDataTypeStr=Inherit: Same as input  ParamDataTypeStr=Inherit: Same as input
  i : Outport
  wires:
  V> pu/1 -> PLL/1(v (pu)), V> pu1/1
  Real-Imag to Complex/1 -> Positive Sequence  current/1(V1(pu))
  PQ/1 -> Demux/1
  Demux/1 -> Real-Imag to Complex1/1
  Demux/2 -> Real-Imag to Complex1/2
  Real-Imag to Complex1/1 -> Positive Sequence  current/2(S_ext)
  Complex to Real-Imag1/1 -> Real-Imag to Complex/1
  Complex to Real-Imag1/2 -> Real-Imag to Complex/2
  Magnitude-Angle to Complex/1 -> Complex to Real-Imag1/1
  Constant/1 -> PLL/2(freq (pu))
  PLL/1(alpha (rad)) -> Magnitude-Angle to Complex/2
  Complex to Magnitude-Angle/2 -> Sum/2
  PLL/2(wt) -> Sum/1
  Sum/1 -> Trigonometric Function1/1
  Trigonometric Function1/1 -> Divide/2
  Complex to Magnitude-Angle/1 -> Divide/1
  RMS1/1 -> IC1/1
  V> pu1/1 -> RMS1/1
  v/1 -> IC2/1
  Positive Sequence  current/1(I1(A)) -> Break  Alg. Loop1/1(In)
  Break  Alg. Loop1/1(Out) -> Complex to Magnitude-Angle/1
  IC1/1 -> Magnitude-Angle to Complex/1
  IC2/1 -> V> pu/1
  Transfer Fcn1/1 -> Gain/1
  Gain/1 -> i/1
  Divide/1 -> Transfer Fcn1/1

== system ng_pv_dynamic_dbus_p_1_sm_ng/SM_NG/Dynamic Load BCDC3/Single-Phase Dynamic Load2/model ==
  v : Inport
  PQ : Inport  Port=2
  Break  Alg. Loop1 : Subsystem
  Complex to Magnitude-Angle : ComplexToMagnitudeAngle
  Complex to Real-Imag1 : ComplexToRealImag
  Constant : Constant
  Demux : Demux  Outputs=2
  Divide : Product  Inputs=**
  Gain : Gain  Gain=1.0114
  IC1 : InitialCondition
  IC2 : InitialCondition
  Magnitude-Angle to Complex : MagnitudeAngleToComplex
  PLL : Subsystem  mask{freq=fnom}
      mask prompts: freq "Initial frequency (Hz)"
  Positive Sequence  current : Subsystem
  RMS1 : powerlib_meascontrol/Measurements/RMS  TrueRMS=on  Freq=fnom  RMSInit=1  Ts=0
  Real-Imag to Complex : RealImagToComplex
  Real-Imag to Complex1 : RealImagToComplex
  Sum : Sum
  Transfer Fcn1 : TransferFcn  Numerator=[1 290.1]  Denominator=[1 298.8]
  Trigonometric Function1 : Trigonometry
  V> pu : Gain  Gain=1/Vbase/sqrt(3)  SaturateOnIntegerOverflow=on  OutDataTypeStr=Inherit: Same as input  ParamDataTypeStr=Inherit: Same as input
  V> pu1 : Gain  Gain=sqrt(2)  SaturateOnIntegerOverflow=on  OutDataTypeStr=Inherit: Same as input  ParamDataTypeStr=Inherit: Same as input
  i : Outport
  wires:
  V> pu/1 -> PLL/1(v (pu)), V> pu1/1
  Real-Imag to Complex/1 -> Positive Sequence  current/1(V1(pu))
  PQ/1 -> Demux/1
  Demux/1 -> Real-Imag to Complex1/1
  Demux/2 -> Real-Imag to Complex1/2
  Real-Imag to Complex1/1 -> Positive Sequence  current/2(S_ext)
  Complex to Real-Imag1/1 -> Real-Imag to Complex/1
  Complex to Real-Imag1/2 -> Real-Imag to Complex/2
  Magnitude-Angle to Complex/1 -> Complex to Real-Imag1/1
  Constant/1 -> PLL/2(freq (pu))
  PLL/1(alpha (rad)) -> Magnitude-Angle to Complex/2
  Complex to Magnitude-Angle/2 -> Sum/2
  PLL/2(wt) -> Sum/1
  Sum/1 -> Trigonometric Function1/1
  Trigonometric Function1/1 -> Divide/2
  Complex to Magnitude-Angle/1 -> Divide/1
  RMS1/1 -> IC1/1
  V> pu1/1 -> RMS1/1
  v/1 -> IC2/1
  Positive Sequence  current/1(I1(A)) -> Break  Alg. Loop1/1(In)
  Break  Alg. Loop1/1(Out) -> Complex to Magnitude-Angle/1
  IC1/1 -> Magnitude-Angle to Complex/1
  IC2/1 -> V> pu/1
  Transfer Fcn1/1 -> Gain/1
  Gain/1 -> i/1
  Divide/1 -> Transfer Fcn1/1

== system ng_pv_dynamic_dbus_p_1_sm_ng/SM_NG/Dynamic Load BCDC3/Single-Phase Dynamic Load9/model ==
  v : Inport
  PQ : Inport  Port=2
  Break  Alg. Loop1 : Subsystem
  Complex to Magnitude-Angle : ComplexToMagnitudeAngle
  Complex to Real-Imag1 : ComplexToRealImag
  Constant : Constant
  Demux : Demux  Outputs=2
  Divide : Product  Inputs=**
  Gain : Gain  Gain=1.0114
  IC1 : InitialCondition
  IC2 : InitialCondition
  Magnitude-Angle to Complex : MagnitudeAngleToComplex
  PLL : Subsystem  mask{freq=fnom}
      mask prompts: freq "Initial frequency (Hz)"
  Positive Sequence  current : Subsystem
  RMS1 : powerlib_meascontrol/Measurements/RMS  TrueRMS=on  Freq=fnom  RMSInit=1  Ts=0
  Real-Imag to Complex : RealImagToComplex
  Real-Imag to Complex1 : RealImagToComplex
  Sum : Sum
  Transfer Fcn1 : TransferFcn  Numerator=[1 290.1]  Denominator=[1 298.8]
  Trigonometric Function1 : Trigonometry
  V> pu : Gain  Gain=1/Vbase/sqrt(3)  SaturateOnIntegerOverflow=on  OutDataTypeStr=Inherit: Same as input  ParamDataTypeStr=Inherit: Same as input
  V> pu1 : Gain  Gain=sqrt(2)  SaturateOnIntegerOverflow=on  OutDataTypeStr=Inherit: Same as input  ParamDataTypeStr=Inherit: Same as input
  i : Outport
  wires:
  V> pu/1 -> PLL/1(v (pu)), V> pu1/1
  Real-Imag to Complex/1 -> Positive Sequence  current/1(V1(pu))
  PQ/1 -> Demux/1
  Demux/1 -> Real-Imag to Complex1/1
  Demux/2 -> Real-Imag to Complex1/2
  Real-Imag to Complex1/1 -> Positive Sequence  current/2(S_ext)
  Complex to Real-Imag1/1 -> Real-Imag to Complex/1
  Complex to Real-Imag1/2 -> Real-Imag to Complex/2
  Magnitude-Angle to Complex/1 -> Complex to Real-Imag1/1
  Constant/1 -> PLL/2(freq (pu))
  PLL/1(alpha (rad)) -> Magnitude-Angle to Complex/2
  Complex to Magnitude-Angle/2 -> Sum/2
  PLL/2(wt) -> Sum/1
  Sum/1 -> Trigonometric Function1/1
  Trigonometric Function1/1 -> Divide/2
  Complex to Magnitude-Angle/1 -> Divide/1
  RMS1/1 -> IC1/1
  V> pu1/1 -> RMS1/1
  v/1 -> IC2/1
  Positive Sequence  current/1(I1(A)) -> Break  Alg. Loop1/1(In)
  Break  Alg. Loop1/1(Out) -> Complex to Magnitude-Angle/1
  IC1/1 -> Magnitude-Angle to Complex/1
  IC2/1 -> V> pu/1
  Transfer Fcn1/1 -> Gain/1
  Gain/1 -> i/1
  Divide/1 -> Transfer Fcn1/1

== system ng_pv_dynamic_dbus_p_1_sm_ng/SM_NG/Single-Phase Dynamic Load30/model/Break  Alg. Loop1 ==
  In : Inport
  Complex to Real-Imag : ComplexToRealImag
  Real-Imag to Complex : RealImagToComplex
  imag : simulink_extras/Additional Linear/Transfer Fcn (with initial outputs)  N=[1]  D="[100e-6  1]"  Y0=imag(I1_init*exp(-j*Pha_V0*pi/180))  U0=imag(I1_init*exp(-j*Pha_V0*pi/180))
  real : simulink_extras/Additional Linear/Transfer Fcn (with initial outputs)  N=[1]  D="[100e-6  1]"  Y0=real(I1_init*exp(-j*Pha_V0*pi/180))  U0=real(I1_init*exp(-j*Pha_V0*pi/180))
  Out : Outport
  wires:
  Complex to Real-Imag/2 -> imag/1
  Complex to Real-Imag/1 -> real/1
  Real-Imag to Complex/1 -> Out/1
  In/1 -> Complex to Real-Imag/1
  imag/1 -> Real-Imag to Complex/2
  real/1 -> Real-Imag to Complex/1

== system ng_pv_dynamic_dbus_p_1_sm_ng/SM_NG/Single-Phase Dynamic Load30/model/PLL ==
  v (pu) : Inport
  freq (pu) : Inport  Port=2
  Gain : Gain  Gain=2*pi
  Gain1 : Gain  Gain=500
  Gain2 : Gain  Gain=freq
  IC : InitialCondition
  Integrator : Integrator
  Integrator1 : Integrator
  Product : Product  Inputs=**  RndMeth=Zero
  Sum1 : Sum  SaturateOnIntegerOverflow=on  InputSameDT=on  OutDataTypeStr=Inherit: Same as first input
  Trigonometric Function : Trigonometry  Operator=cos
  adaptive filter : Subsystem
  adaptive mean : Subsystem
  alpha (rad) : Outport
  wt : Outport  Port=2
  wires:
  freq (pu)/1 -> Gain2/1
  Gain2/1 -> adaptive filter/2(freq (Hz)), adaptive mean/2(freq (Hz)), Gain/1
  Trigonometric Function/1 -> Product/2
  adaptive mean/1(y) -> alpha (rad)/1
  Integrator1/1 -> Gain1/1
  Gain1/1 -> Sum1/1, adaptive mean/1(u)
  Sum1/1 -> Trigonometric Function/1
  Integrator/1 -> Sum1/2, wt/1
  Gain/1 -> Integrator/1
  adaptive filter/1(y) -> Integrator1/1
  Product/1 -> adaptive filter/1(u)
  v (pu)/1 -> IC/1
  IC/1 -> Product/1

== system ng_pv_dynamic_dbus_p_1_sm_ng/SM_NG/Single-Phase Dynamic Load30/model/Positive Sequence  current ==
  note: I1= (S/V1)'
  V1(pu) : Inport
  S_ext : Inport  Port=2
  Conj1 : Math  Operator=conj  SaturateOnIntegerOverflow=on
  Product : Product  Inputs=/*  SaturateOnIntegerOverflow=on  InputSameDT=on  OutDataTypeStr=Inherit: Same as first input
  pu>V : Gain  Gain=Vnom/sqrt(2)  SaturateOnIntegerOverflow=on  OutDataTypeStr=Inherit: Same as input  ParamDataTypeStr=Inherit: Same as input
  I1(A) : Outport
  wires:
  V1(pu)/1 -> pu>V/1
  Product/1 -> Conj1/1
  Conj1/1 -> I1(A)/1
  S_ext/1 -> Product/2
  pu>V/1 -> Product/1

== system ng_pv_dynamic_dbus_p_1_sm_ng/SM_NG/Single-Phase Dynamic Load32/model/Break  Alg. Loop1 ==
  In : Inport
  Complex to Real-Imag : ComplexToRealImag
  Real-Imag to Complex : RealImagToComplex
  imag : simulink_extras/Additional Linear/Transfer Fcn (with initial outputs)  N=[1]  D="[100e-6  1]"  Y0=imag(I1_init*exp(-j*Pha_V0*pi/180))  U0=imag(I1_init*exp(-j*Pha_V0*pi/180))
  real : simulink_extras/Additional Linear/Transfer Fcn (with initial outputs)  N=[1]  D="[100e-6  1]"  Y0=real(I1_init*exp(-j*Pha_V0*pi/180))  U0=real(I1_init*exp(-j*Pha_V0*pi/180))
  Out : Outport
  wires:
  Complex to Real-Imag/2 -> imag/1
  Complex to Real-Imag/1 -> real/1
  Real-Imag to Complex/1 -> Out/1
  In/1 -> Complex to Real-Imag/1
  imag/1 -> Real-Imag to Complex/2
  real/1 -> Real-Imag to Complex/1

== system ng_pv_dynamic_dbus_p_1_sm_ng/SM_NG/Single-Phase Dynamic Load32/model/PLL ==
  v (pu) : Inport
  freq (pu) : Inport  Port=2
  Gain : Gain  Gain=2*pi
  Gain1 : Gain  Gain=500
  Gain2 : Gain  Gain=freq
  IC : InitialCondition
  Integrator : Integrator
  Integrator1 : Integrator
  Product : Product  Inputs=**  RndMeth=Zero
  Sum1 : Sum  SaturateOnIntegerOverflow=on  InputSameDT=on  OutDataTypeStr=Inherit: Same as first input
  Trigonometric Function : Trigonometry  Operator=cos
  adaptive filter : Subsystem
  adaptive mean : Subsystem
  alpha (rad) : Outport
  wt : Outport  Port=2
  wires:
  freq (pu)/1 -> Gain2/1
  Gain2/1 -> adaptive filter/2(freq (Hz)), adaptive mean/2(freq (Hz)), Gain/1
  Trigonometric Function/1 -> Product/2
  adaptive mean/1(y) -> alpha (rad)/1
  Integrator1/1 -> Gain1/1
  Gain1/1 -> Sum1/1, adaptive mean/1(u)
  Sum1/1 -> Trigonometric Function/1
  Integrator/1 -> Sum1/2, wt/1
  Gain/1 -> Integrator/1
  adaptive filter/1(y) -> Integrator1/1
  Product/1 -> adaptive filter/1(u)
  v (pu)/1 -> IC/1
  IC/1 -> Product/1

== system ng_pv_dynamic_dbus_p_1_sm_ng/SM_NG/Single-Phase Dynamic Load32/model/Positive Sequence  current ==
  note: I1= (S/V1)'
  V1(pu) : Inport
  S_ext : Inport  Port=2
  Conj1 : Math  Operator=conj  SaturateOnIntegerOverflow=on
  Product : Product  Inputs=/*  SaturateOnIntegerOverflow=on  InputSameDT=on  OutDataTypeStr=Inherit: Same as first input
  pu>V : Gain  Gain=Vnom/sqrt(2)  SaturateOnIntegerOverflow=on  OutDataTypeStr=Inherit: Same as input  ParamDataTypeStr=Inherit: Same as input
  I1(A) : Outport
  wires:
  V1(pu)/1 -> pu>V/1
  Product/1 -> Conj1/1
  Conj1/1 -> I1(A)/1
  S_ext/1 -> Product/2
  pu>V/1 -> Product/1

== system ng_pv_dynamic_dbus_p_1_sm_ng/SM_NG/Single-Phase Dynamic Load33/model/Break  Alg. Loop1 ==
  In : Inport
  Complex to Real-Imag : ComplexToRealImag
  Real-Imag to Complex : RealImagToComplex
  imag : simulink_extras/Additional Linear/Transfer Fcn (with initial outputs)  N=[1]  D="[100e-6  1]"  Y0=imag(I1_init*exp(-j*Pha_V0*pi/180))  U0=imag(I1_init*exp(-j*Pha_V0*pi/180))
  real : simulink_extras/Additional Linear/Transfer Fcn (with initial outputs)  N=[1]  D="[100e-6  1]"  Y0=real(I1_init*exp(-j*Pha_V0*pi/180))  U0=real(I1_init*exp(-j*Pha_V0*pi/180))
  Out : Outport
  wires:
  Complex to Real-Imag/2 -> imag/1
  Complex to Real-Imag/1 -> real/1
  Real-Imag to Complex/1 -> Out/1
  In/1 -> Complex to Real-Imag/1
  imag/1 -> Real-Imag to Complex/2
  real/1 -> Real-Imag to Complex/1

== system ng_pv_dynamic_dbus_p_1_sm_ng/SM_NG/Single-Phase Dynamic Load33/model/PLL ==
  v (pu) : Inport
  freq (pu) : Inport  Port=2
  Gain : Gain  Gain=2*pi
  Gain1 : Gain  Gain=500
  Gain2 : Gain  Gain=freq
  IC : InitialCondition
  Integrator : Integrator
  Integrator1 : Integrator
  Product : Product  Inputs=**  RndMeth=Zero
  Sum1 : Sum  SaturateOnIntegerOverflow=on  InputSameDT=on  OutDataTypeStr=Inherit: Same as first input
  Trigonometric Function : Trigonometry  Operator=cos
  adaptive filter : Subsystem
  adaptive mean : Subsystem
  alpha (rad) : Outport
  wt : Outport  Port=2
  wires:
  freq (pu)/1 -> Gain2/1
  Gain2/1 -> adaptive filter/2(freq (Hz)), adaptive mean/2(freq (Hz)), Gain/1
  Trigonometric Function/1 -> Product/2
  adaptive mean/1(y) -> alpha (rad)/1
  Integrator1/1 -> Gain1/1
  Gain1/1 -> Sum1/1, adaptive mean/1(u)
  Sum1/1 -> Trigonometric Function/1
  Integrator/1 -> Sum1/2, wt/1
  Gain/1 -> Integrator/1
  adaptive filter/1(y) -> Integrator1/1
  Product/1 -> adaptive filter/1(u)
  v (pu)/1 -> IC/1
  IC/1 -> Product/1

== system ng_pv_dynamic_dbus_p_1_sm_ng/SM_NG/Single-Phase Dynamic Load33/model/Positive Sequence  current ==
  note: I1= (S/V1)'
  V1(pu) : Inport
  S_ext : Inport  Port=2
  Conj1 : Math  Operator=conj  SaturateOnIntegerOverflow=on
  Product : Product  Inputs=/*  SaturateOnIntegerOverflow=on  InputSameDT=on  OutDataTypeStr=Inherit: Same as first input
  pu>V : Gain  Gain=Vnom/sqrt(2)  SaturateOnIntegerOverflow=on  OutDataTypeStr=Inherit: Same as input  ParamDataTypeStr=Inherit: Same as input
  I1(A) : Outport
  wires:
  V1(pu)/1 -> pu>V/1
  Product/1 -> Conj1/1
  Conj1/1 -> I1(A)/1
  S_ext/1 -> Product/2
  pu>V/1 -> Product/1

== system ng_pv_dynamic_dbus_p_1_sm_ng/SM_NG/Single-Phase Dynamic Load34/model/Break  Alg. Loop1 ==
  In : Inport
  Complex to Real-Imag : ComplexToRealImag
  Real-Imag to Complex : RealImagToComplex
  imag : simulink_extras/Additional Linear/Transfer Fcn (with initial outputs)  N=[1]  D="[100e-6  1]"  Y0=imag(I1_init*exp(-j*Pha_V0*pi/180))  U0=imag(I1_init*exp(-j*Pha_V0*pi/180))
  real : simulink_extras/Additional Linear/Transfer Fcn (with initial outputs)  N=[1]  D="[100e-6  1]"  Y0=real(I1_init*exp(-j*Pha_V0*pi/180))  U0=real(I1_init*exp(-j*Pha_V0*pi/180))
  Out : Outport
  wires:
  Complex to Real-Imag/2 -> imag/1
  Complex to Real-Imag/1 -> real/1
  Real-Imag to Complex/1 -> Out/1
  In/1 -> Complex to Real-Imag/1
  imag/1 -> Real-Imag to Complex/2
  real/1 -> Real-Imag to Complex/1

== system ng_pv_dynamic_dbus_p_1_sm_ng/SM_NG/Single-Phase Dynamic Load34/model/PLL ==
  v (pu) : Inport
  freq (pu) : Inport  Port=2
  Gain : Gain  Gain=2*pi
  Gain1 : Gain  Gain=500
  Gain2 : Gain  Gain=freq
  IC : InitialCondition
  Integrator : Integrator
  Integrator1 : Integrator
  Product : Product  Inputs=**  RndMeth=Zero
  Sum1 : Sum  SaturateOnIntegerOverflow=on  InputSameDT=on  OutDataTypeStr=Inherit: Same as first input
  Trigonometric Function : Trigonometry  Operator=cos
  adaptive filter : Subsystem
  adaptive mean : Subsystem
  alpha (rad) : Outport
  wt : Outport  Port=2
  wires:
  freq (pu)/1 -> Gain2/1
  Gain2/1 -> adaptive filter/2(freq (Hz)), adaptive mean/2(freq (Hz)), Gain/1
  Trigonometric Function/1 -> Product/2
  adaptive mean/1(y) -> alpha (rad)/1
  Integrator1/1 -> Gain1/1
  Gain1/1 -> Sum1/1, adaptive mean/1(u)
  Sum1/1 -> Trigonometric Function/1
  Integrator/1 -> Sum1/2, wt/1
  Gain/1 -> Integrator/1
  adaptive filter/1(y) -> Integrator1/1
  Product/1 -> adaptive filter/1(u)
  v (pu)/1 -> IC/1
  IC/1 -> Product/1

== system ng_pv_dynamic_dbus_p_1_sm_ng/SM_NG/Single-Phase Dynamic Load34/model/Positive Sequence  current ==
  note: I1= (S/V1)'
  V1(pu) : Inport
  S_ext : Inport  Port=2
  Conj1 : Math  Operator=conj  SaturateOnIntegerOverflow=on
  Product : Product  Inputs=/*  SaturateOnIntegerOverflow=on  InputSameDT=on  OutDataTypeStr=Inherit: Same as first input
  pu>V : Gain  Gain=Vnom/sqrt(2)  SaturateOnIntegerOverflow=on  OutDataTypeStr=Inherit: Same as input  ParamDataTypeStr=Inherit: Same as input
  I1(A) : Outport
  wires:
  V1(pu)/1 -> pu>V/1
  Product/1 -> Conj1/1
  Conj1/1 -> I1(A)/1
  S_ext/1 -> Product/2
  pu>V/1 -> Product/1

== system ng_pv_dynamic_dbus_p_1_sm_ng/SM_NG/Single-Phase Dynamic Load35/model/Break  Alg. Loop ==
  In : Inport
  Complex to Real-Imag : ComplexToRealImag
  Real-Imag to Complex : RealImagToComplex
  imag : simulink_extras/Additional Linear/Transfer Fcn (with initial outputs)  N=[1]  D="[1000e-6  1]"  Y0=imag(I1_init*exp(-j*Pha_V0*pi/180))  U0=imag(I1_init*exp(-j*Pha_V0*pi/180))
  real : simulink_extras/Additional Linear/Transfer Fcn (with initial outputs)  N=[1]  D="[1000e-6  1]"  Y0=real(I1_init*exp(-j*Pha_V0*pi/180))  U0=real(I1_init*exp(-j*Pha_V0*pi/180))
  Out : Outport
  wires:
  imag/1 -> Real-Imag to Complex/2
  Complex to Real-Imag/2 -> imag/1
  real/1 -> Real-Imag to Complex/1
  Complex to Real-Imag/1 -> real/1
  Real-Imag to Complex/1 -> Out/1
  In/1 -> Complex to Real-Imag/1

== system ng_pv_dynamic_dbus_p_1_sm_ng/SM_NG/Single-Phase Dynamic Load35/model/PLL ==
  v (pu) : Inport
  freq (pu) : Inport  Port=2
  Gain : Gain  Gain=2*pi
  Gain1 : Gain  Gain=500
  Gain2 : Gain  Gain=freq
  IC : InitialCondition
  Integrator : Integrator
  Integrator1 : Integrator
  Product : Product  Inputs=**  RndMeth=Zero
  Sum1 : Sum  SaturateOnIntegerOverflow=on  InputSameDT=on  OutDataTypeStr=Inherit: Same as first input
  Trigonometric Function : Trigonometry  Operator=cos
  adaptive filter : Subsystem
  adaptive mean : Subsystem
  alpha (rad) : Outport
  wt : Outport  Port=2
  wires:
  freq (pu)/1 -> Gain2/1
  Gain2/1 -> adaptive filter/2(freq (Hz)), adaptive mean/2(freq (Hz)), Gain/1
  Trigonometric Function/1 -> Product/2
  adaptive mean/1(y) -> alpha (rad)/1
  Integrator1/1 -> Gain1/1
  Gain1/1 -> Sum1/1, adaptive mean/1(u)
  Sum1/1 -> Trigonometric Function/1
  Integrator/1 -> Sum1/2, wt/1
  Gain/1 -> Integrator/1
  adaptive filter/1(y) -> Integrator1/1
  Product/1 -> adaptive filter/1(u)
  v (pu)/1 -> IC/1
  IC/1 -> Product/1

== system ng_pv_dynamic_dbus_p_1_sm_ng/SM_NG/Single-Phase Dynamic Load35/model/Positive Sequence  current ==
  note: I1= (S/V1)'
  V1(pu) : Inport
  S_ext : Inport  Port=2
  Conj1 : Math  Operator=conj  SaturateOnIntegerOverflow=on
  Product : Product  Inputs=/*  SaturateOnIntegerOverflow=on  InputSameDT=on  OutDataTypeStr=Inherit: Same as first input
  pu>V : Gain  Gain=Vnom/sqrt(2)  SaturateOnIntegerOverflow=on  OutDataTypeStr=Inherit: Same as input  ParamDataTypeStr=Inherit: Same as input
  I1(A) : Outport
  wires:
  V1(pu)/1 -> pu>V/1
  Product/1 -> Conj1/1
  Conj1/1 -> I1(A)/1
  S_ext/1 -> Product/2
  pu>V/1 -> Product/1
